simulink model "Auris_Desaturation"  (R2019a)
settings: Solver=FixedStepAuto  StartTime=0.0  StopTime=1000  FixedStep=.1  RelTol=1e-5
PostLoadFcn:
  | if builtin('license','test','virtual_reality_toolbox')
  |     set_param([gcs '/Simulink 3D Animation'], 'enableVis', 'on')
  | else
  |     set_param([gcs '/Simulink 3D Animation'], 'enableVis', 'off')
  | end
InitFcn:
  | if strcmp(get_param([gcs '/Simulink 3D Animation'], 'enableVis'), 'on')
  |     if ~builtin('license','checkout','virtual_reality_toolbox')
  |         error(message('aeroblks_cubesat:cubesat:licenseFailAnimTemplate'));
  |     end
  | end
model workspace (MATLAB code in the model file + MAT data in the model file):
  aeroCoeff : struct (value not decoded)
  environment : struct (value not decoded)
  initCond : struct (value not decoded)
  inputs0 : struct (value not decoded)
  states0 : struct (value not decoded)
  vehicle : struct (value not decoded)
  other statements: initialize6DOFSkyHogg;
values from neighbouring files (symbols this model uses):
  epoch = juliandate(tle.epoch.year, 1, 1) + tle.epoch.day * 86400    [ADC_Sim_init.m]
  inertia = inertia * conversion    [ADC_Sim_init.m]
  initial_ang_rate = [15, 15, 15]    [ADC_Sim_init.m]
  initial_euler = [74, 36, 33]    [ADC_Sim_init.m]
  magnetic_dipole = 0.66    [ADC_Sim_init.m]
  semi_major = (((86400 / tle.mean_motion) / (2 * pi))^2 * 398.6e12)^(1 / 3)    [ADC_Sim_init.m]
  starting_time = juliandate(date)    [ADC_Sim_init.m]
  tle = read_tloes('ISS_TLE.txt')    [ADC_Sim_init.m]
  true_anomaly = tle.mean_anomaly + (2 * exp(1) - 1 / 4 * exp(3)) * sind(tle.mean_anomaly) + 5 / 4 * exp(2) * sind(2 * tle.mean_anomaly) + 13/12 * exp(3) * sind(3 * tle.mean_anomaly)    [ADC_Sim_init.m]
undefined symbols (not defined in the file or in its folder): Earth, euler0, IAU, km, pqr0, s, WGS84
libraries: aerolibutil x19, vrlib x12, aerolibconvert2 x5, sharedtransform x4, aerolibtransform2 x4, aerolibgravity2 x2, aerolibcelestial x2, aerolib6dof2 x1, dspmtrx3 x1, sharedutil x1, simulink_extras x1, aerolibobsolete x1
(part 2 of 2)

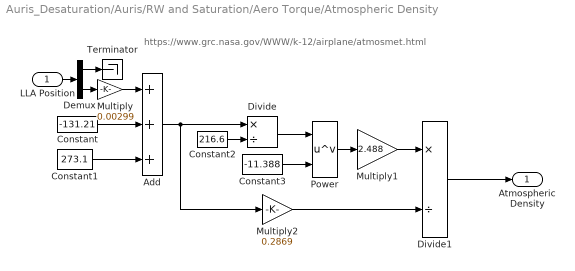
== system Auris_Desaturation/Auris/RW and Saturation/Aero Torque/Atmospheric Density ==
  note: https://www.grc.nasa.gov/WWW/k-12/airplane/atmosmet.html
  LLA Position : Inport
  Add : Sum  Inputs=+++
  Constant : Constant  Value=-131.21
  Constant1 : Constant  Value=273.1
  Constant2 : Constant  Value=216.6
  Constant3 : Constant  Value=-11.388
  Demux : Demux  Outputs=2
  Divide : Product  Inputs=*/
  Divide1 : Product  Inputs=*/
  Multiply : Gain  Gain=0.00299
  Multiply1 : Gain  Gain=2.488
  Multiply2 : Gain  Gain=0.2869
  Power : Math  Operator=pow  SaturateOnIntegerOverflow=on
  Terminator : Terminator
  Atmospheric Density : Outport
  wires:
  LLA Position/1 -> Demux/1
  Demux/1 -> Terminator/1
  Constant/1 -> Add/2
  Multiply/1 -> Add/1
  Demux/2 -> Multiply/1
  Constant1/1 -> Add/3
  Add/1 -> Multiply2/1, Divide/1
  Constant2/1 -> Divide/2
  Divide/1 -> Power/1
  Constant3/1 -> Power/2
  Power/1 -> Multiply1/1
  Multiply1/1 -> Divide1/1
  Multiply2/1 -> Divide1/2
  Divide1/1 -> Atmospheric Density/1

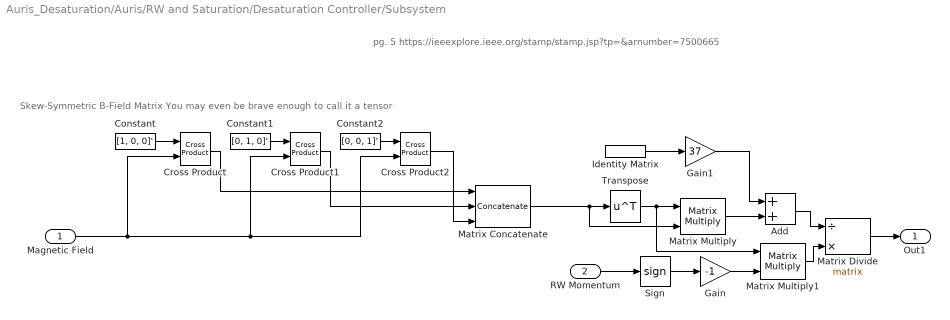
== system Auris_Desaturation/Auris/RW and Saturation/Desaturation Controller/Subsystem ==
  note: pg. 5 https://ieeexplore.ieee.org/stamp/stamp.jsp?tp=&arnumber=7500665
  note: Skew-Symmetric B-Field Matrix
      | You may even be brave enough to call it a tensor
  Magnetic Field : Inport
  RW Momentum : Inport  Port=2
  Add : Sum
  Constant : Constant  Value=[1, 0, 0]'
  Constant1 : Constant  Value=[0, 1, 0]'
  Constant2 : Constant  Value=[0, 0, 1]'
  Cross Product : vrlib/Utilities/Cross Product
      settings: SourceProductName=Simulink
  Cross Product1 : vrlib/Utilities/Cross Product
      settings: SourceProductName=Simulink
  Cross Product2 : vrlib/Utilities/Cross Product
      settings: SourceProductName=Simulink
  Gain : Gain  Gain=-1
  Gain1 : Gain  Gain=37
  Identity Matrix : dspmtrx3/Identity Matrix  Inherit=off  N=3  Ts=1  dataType=double  isSigned=on  wordLen=16  udDataType=sfix(16)  fracBitsMode=Best precision  numFracBits=15  OutDataTypeStr=double  LastOutDataTypeStr=double
      settings: SourceProductName=DSP System Toolbox
  Matrix Concatenate : Concatenate  NumInputs=3  Mode=Multidimensional array  ConcatenateDimension=2
  Matrix Divide : Product  Inputs=/*  Multiplication=Matrix(*)
  Matrix Multiply : Product  Multiplication=Matrix(*)
  Matrix Multiply1 : Product  Multiplication=Matrix(*)
  Sign : Signum
  Transpose : Math  Operator=transpose  SaturateOnIntegerOverflow=on
  Out1 : Outport
  wires:
  Constant/1 -> Cross Product/1
  Constant1/1 -> Cross Product1/1
  Constant2/1 -> Cross Product2/1
  Magnetic Field/1 -> Cross Product2/2, Cross Product1/2, Cross Product/2
  Cross Product/1 -> Matrix Concatenate/1
  Cross Product1/1 -> Matrix Concatenate/2
  Cross Product2/1 -> Matrix Concatenate/3
  Matrix Concatenate/1 -> Matrix Multiply/2, Transpose/1
  Transpose/1 -> Matrix Multiply1/1, Matrix Multiply/1
  Matrix Multiply/1 -> Add/2
  Identity Matrix/1 -> Gain1/1
  Sign/1 -> Gain/1
  RW Momentum/1 -> Sign/1
  Gain/1 -> Matrix Multiply1/2
  Matrix Multiply1/1 -> Matrix Divide/2
  Add/1 -> Matrix Divide/1
  Matrix Divide/1 -> Out1/1
  Gain1/1 -> Add/1
